simulink model "OtterFullModel"  (R2020b)
settings: Solver=VariableStepAuto  StartTime=0.0  StopTime=20  RelTol=1e-3
libraries: simulink x1, mssSimulink x1
settings Model: Creator=rapha  LastModifiedBy=rapha

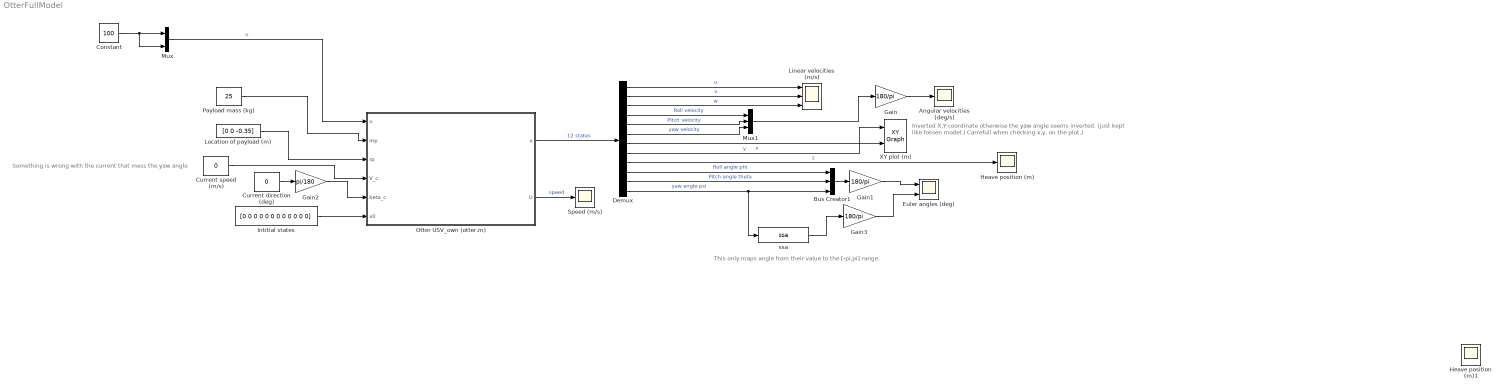
== system OtterFullModel ==
  note: Inverted X,Y coordinate otherwise the yaw angle seems inverted.
      | (just kept like fossen model.) Carrefull when checking x,y, on the plot.)
  note: This only maps angle from their value to the [-pi,pi] range.
  note: Something is wrong with the current that mess the yaw angle
  Angular velocities (deg/s) : Scope
  Bus Creator1 : BusCreator  Inputs=3
  Constant : Constant  Value=100
  Current direction (deg) : Constant  Value=0
  Current speed (m/s) : Constant  Value=0
  Demux : Demux  Outputs=12
  Euler angles (deg) : Scope  NumInputPorts=2
  Gain : Gain  Gain=180/pi
  Gain1 : Gain  Gain=180/pi
  Gain2 : Gain  Gain=pi/180
  Gain3 : Gain  Gain=180/pi
  Heave position (m) : Scope
  Heave position (m)1 : Scope
  Intitial states : Constant  Value=[0 0 0 0 0 0 0 0 0 0 0 0]
  Linear velocities (m/s) : Scope  NumInputPorts=3
  Location of payload (m) : Constant  Value=[0 0 -0.35]
  Mux : Mux  Inputs=2
  Mux1 : Mux  Inputs=3
  "Otter USV_own (otter.m) " : Subsystem  AncestorBlock=mssSimulink/Marine craft models/Otter USV (otter.m)
      mask Display: image('otter.jpg'); % Use "Edit Image" on toolstrip to change.
  Payload mass (kg) : Constant  Value=25
  Speed (m/s) : Scope
  XY plot (m) : simulink/Sinks/XY Graph  xmin=-70  xmax=70  ymin=-70  ymax=70  st=0.01
  "ssa   " : mssSimulink/Utilities/Math Operations/ssa  SystemSampleTime=-1  VariantActivationTime=update diagram  Latency=0  AutoFrameSizeCalculation=off
  wires:
  "Otter USV_own (otter.m) "/1(x) -> Demux/1  "12 states"
  Intitial states/1 -> "Otter USV_own (otter.m) "/6(x0)
  Payload mass (kg)/1 -> "Otter USV_own (otter.m) "/2(mp)
  Gain2/1 -> "Otter USV_own (otter.m) "/5(beta_c)
  Mux/1 -> "Otter USV_own (otter.m) "/1(n)  "n"
  Current direction (deg)/1 -> Gain2/1
  "Otter USV_own (otter.m) "/2(U) -> Speed (m/s)/1  "speed"
  Current speed (m/s)/1 -> "Otter USV_own (otter.m) "/4(V_c)
  Location of payload (m)/1 -> "Otter USV_own (otter.m) "/3(rp)
  Demux/1 -> Linear velocities (m/s)/1  "u"
  Demux/8 -> XY plot (m)/1  "y"
  Demux/7 -> XY plot (m)/2  "x"
  Demux/2 -> Linear velocities (m/s)/2  "v"
  Demux/3 -> Linear velocities (m/s)/3  "w"
  Gain/1 -> Angular velocities (deg/s)/1
  Mux1/1 -> Gain/1
  Demux/4 -> Mux1/1  "Roll velocity"
  Demux/5 -> Mux1/2  "Pitch velocity"
  Demux/6 -> Mux1/3  "yaw velocity"
  Demux/9 -> Heave position (m)/1  "z"
  Demux/11 -> Bus Creator1/2  "Pitch angle theta"
  Gain1/1 -> Euler angles (deg)/1
  Bus Creator1/1 -> Gain1/1
  Demux/10 -> Bus Creator1/1  "Roll angle phi"
  Demux/12 -> "ssa   "/1, Bus Creator1/3  "yaw angle psi"
  Constant/1 -> Mux/2, Mux/1
  "ssa   "/1 -> Gain3/1
  Gain3/1 -> Euler angles (deg)/2

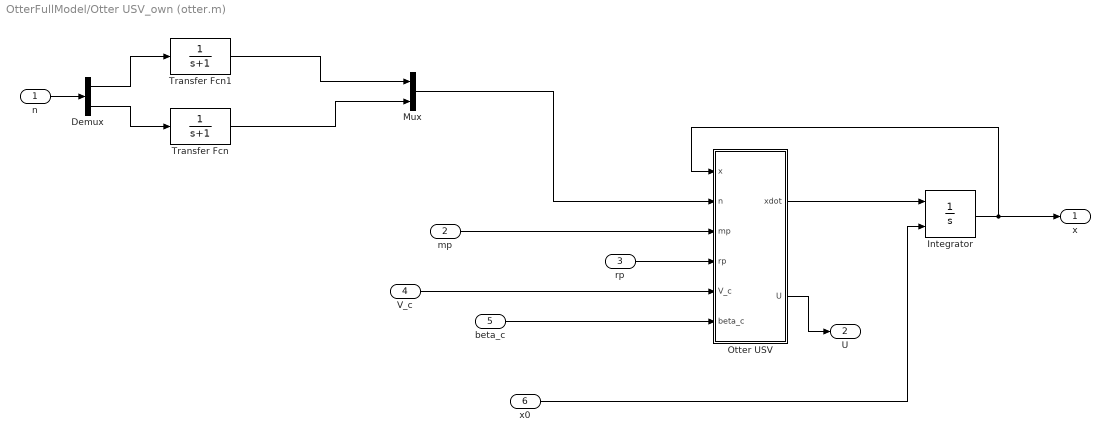
== system OtterFullModel/Otter USV_own (otter.m)  ==
  n : Inport
  mp : Inport  Port=2
  rp : Inport  Port=3
  V_c : Inport  Port=4
  beta_c : Inport  Port=5
  x0 : Inport  Port=6
  Demux : Demux  Outputs=2
  Integrator : Integrator  InitialConditionSource=external  InitialCondition=[1 1]  UpperSaturationLimit=10  LowerSaturationLimit=-10  AbsoluteTolerance=1e-3
  Mux : Mux  Inputs=2
  Otter USV : MATLAB Function  TreatAsAtomicUnit=on
  Transfer Fcn : TransferFcn  Denominator=[1 1]
  Transfer Fcn1 : TransferFcn  Denominator=[1 1]
  x : Outport
  U : Outport  Port=2
  wires:
  Transfer Fcn1/1 -> Mux/1
  Transfer Fcn/1 -> Mux/2
  V_c/1 -> Otter USV/5(V_c)
  Otter USV/2(U) -> U/1
  mp/1 -> Otter USV/3(mp)
  Otter USV/1(xdot) -> Integrator/1
  Integrator/1 -> Otter USV/1(x), x/1
  beta_c/1 -> Otter USV/6(beta_c)
  rp/1 -> Otter USV/4(rp)
  x0/1 -> Integrator/2
  Demux/1 -> Transfer Fcn1/1
  Demux/2 -> Transfer Fcn/1
  n/1 -> Demux/1
  Mux/1 -> Otter USV/2(n)

== matlab function OtterFullModel/Otter USV_own (otter.m) /Otter USV ==
  settings: updateMethod=DISCRETE
  data: x input; n input; xdot output; mp input; rp input; V_c input; beta_c input; U output
function [xdot, U] = fcn(x,n,mp,rp,V_c,beta_c)

[xdot,U] = OtterFunction(x,n,mp,rp,V_c,beta_c);

end
